simulink model "event"  (R2020a)
settings: Solver=VariableStepAuto  StartTime=0.0  StopTime=5  RelTol=1e-3
settings Model: Creator=I3  LastModifiedBy=I3

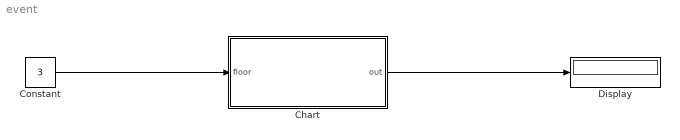
== system event ==
  Chart : Stateflow chart  TreatAsAtomicUnit=on
  Constant : Constant  Value=3
  Display : Display
  wires:
  Constant/1 -> Chart/1(floor)
  Chart/1(out) -> Display/1

== stateflow chart event/Chart ==
  state active
    state stop
      out=current;
    state down
      entry:
      current=0;
      du:
      current=current-1;
    state up
      entry:
      current=0;
      du:
      current=current+1;
    stop -> stop [order 1] : [floor==current]
    (default) -> stop
    stop -> up [order 2] : [current<floor]/{send(up,floor_c)}
    stop -> down [order 3] : [current>floor]/{send(down,floor_c)}
    up -> stop : [current==floor]
    down -> stop : [current==floor]
  state floor_c
    state s2
      entry:
      out=2;
    state s3
      entry:
      out=3;
      current=out;
    state s4
      entry:
      out=4;
    state s1
      entry:
      current=1;
      out=1;
    state s5
      entry:
      out=5;
    (default) -> s1
    s4 -> s3 [order 2] : down
    s4 -> s5 [order 1] : up
    s2 -> s3 [order 1] : up
    s1 -> s2 : up
    s3 -> s2 [order 2] : down
    s3 -> s4 [order 1] : up
    s2 -> s1 [order 2] : down
    s5 -> s4 : down
  (default) -> active
  data: out output; current local =0; floor input
  events: down local FUNCTION_CALL_EVENT; up local FUNCTION_CALL_EVENT
